simulink subsystem "From_relay_board"  (R2021b)
settings: Solver=VariableStepAuto  StartTime=0.0  StopTime=10.0  RelTol=1e-3
libraries: rti1401lib_dio_type4 x3, rtican x1
settings Model: Creator=tsuyoshi  LastModifiedBy=tsuyoshi

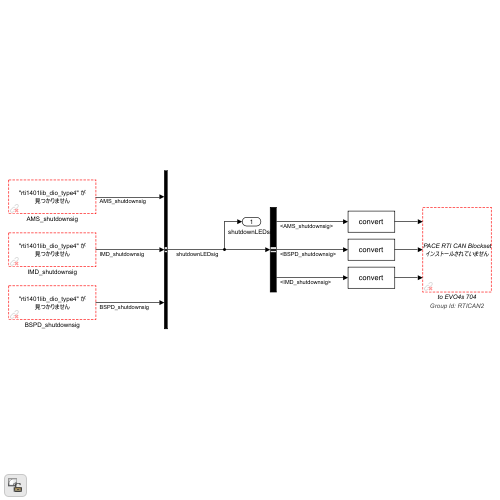
[thumbnail: Simulink's stored preview of the top-level diagram]
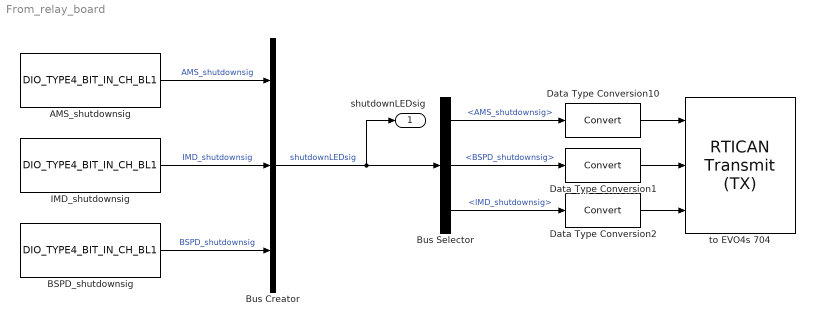
== system From_relay_board ==
  AMS_shutdownsig : rti1401lib_dio_type4/DIO_TYPE4_BIT_IN_CH_BL1  DSProperties=struct('RTI',struct('Version',uint32(1),'BlockType',struct('isSLSource',uint8(1),'isSLSink',uint8(0),'isHWSource',uint8(1),'isHWSink',uint8(0),'isSetup',uint8(0),'isInline',uint8(1),'isNonInline',uint8(0),'isInterrupt',uint8(0),'isChannelwise',uint8(1)),'IOBoardType',{{'DS1401','STD','DIOT4'}},'UnitType','BIT','Identifier','BITINCH','DialogType','ML','BlockSet','NONE','SlaveProcessor','NONE'))  RTIBlockInterface=struct('OutputPortsWidth',int32(1),'OutputPortsDataType',{{'SS_BOOLEAN'}},'OutputPortsActive',1,'OutputPortsName',{{'Out'}},'BlockDisplay',{{['DIO TP4 BIT IN\n Channelwise\nModule: 1\nPort: 1\nChannel: 5'],'center'}},'IconTransparency','on','InitLevel',3,'DialogFcn','rti1401stddiot4bitinchgui','BlockName',struct('Token',{{'DIO_TYPE4_BIT_IN_CH_BL1'}}))  RTIBlockParameters=struct('ModuleNo',{{1,'OFF',[1 16]}},'PortNo',{{1,'OFF',[1 2]}},'ChannelNo',{{5,'OFF',[1 16]}},'TLCFileName',{{'rti1401dio_t4_bit_in_ch','OFF',[]}},'EnableInterrupt',{{0,'OFF',[0 1]}},'TriggerEdgeType',{{1,'OFF',[1 3]}})  RTISFcnParameters=struct('ModuleNo','int32','PortNo','int16','ChannelNo','int16','TLCFileName','char','EnableInterrupt','int16','TriggerEdgeType','int32')  RTIBlockParaDefault=struct('ModuleNo',1,'PortNo',1,'ChannelNo',1,'TLCFileName','rti1401dio_t4_bit_in_ch','EnableInterrupt',0,'TriggerEdgeType',1)
  BSPD_shutdownsig : rti1401lib_dio_type4/DIO_TYPE4_BIT_IN_CH_BL1  DSProperties=struct('RTI',struct('Version',uint32(1),'BlockType',struct('isSLSource',uint8(1),'isSLSink',uint8(0),'isHWSource',uint8(1),'isHWSink',uint8(0),'isSetup',uint8(0),'isInline',uint8(1),'isNonInline',uint8(0),'isInterrupt',uint8(0),'isChannelwise',uint8(1)),'IOBoardType',{{'DS1401','STD','DIOT4'}},'UnitType','BIT','Identifier','BITINCH','DialogType','ML','BlockSet','NONE','SlaveProcessor','NONE'))  RTIBlockInterface=struct('OutputPortsWidth',int32(1),'OutputPortsDataType',{{'SS_BOOLEAN'}},'OutputPortsActive',1,'OutputPortsName',{{'Out'}},'BlockDisplay',{{['DIO TP4 BIT IN\n Channelwise\nModule: 1\nPort: 1\nChannel: 15'],'center'}},'IconTransparency','on','InitLevel',3,'DialogFcn','rti1401stddiot4bitinchgui','BlockName',struct('Token',{{'DIO_TYPE4_BIT_IN_CH_BL1'}}))  RTIBlockParameters=struct('ModuleNo',{{1,'OFF',[1 16]}},'PortNo',{{1,'OFF',[1 2]}},'ChannelNo',{{15,'OFF',[1 16]}},'TLCFileName',{{'rti1401dio_t4_bit_in_ch','OFF',[]}},'EnableInterrupt',{{0,'OFF',[0 1]}},'TriggerEdgeType',{{1,'OFF',[1 3]}})  RTISFcnParameters=struct('ModuleNo','int32','PortNo','int16','ChannelNo','int16','TLCFileName','char','EnableInterrupt','int16','TriggerEdgeType','int32')  RTIBlockParaDefault=struct('ModuleNo',1,'PortNo',1,'ChannelNo',1,'TLCFileName','rti1401dio_t4_bit_in_ch','EnableInterrupt',0,'TriggerEdgeType',1)
  Bus Creator : BusCreator  Inputs=3
  Bus Selector : BusSelector  OutputSignals=AMS_shutdownsig,BSPD_shutdownsig,IMD_shutdownsig
  Data Type Conversion1 : DataTypeConversion
  Data Type Conversion10 : DataTypeConversion
  Data Type Conversion2 : DataTypeConversion
  IMD_shutdownsig : rti1401lib_dio_type4/DIO_TYPE4_BIT_IN_CH_BL1  DSProperties=struct('RTI',struct('Version',uint32(1),'BlockType',struct('isSLSource',uint8(1),'isSLSink',uint8(0),'isHWSource',uint8(1),'isHWSink',uint8(0),'isSetup',uint8(0),'isInline',uint8(1),'isNonInline',uint8(0),'isInterrupt',uint8(0),'isChannelwise',uint8(1)),'IOBoardType',{{'DS1401','STD','DIOT4'}},'UnitType','BIT','Identifier','BITINCH','DialogType','ML','BlockSet','NONE','SlaveProcessor','NONE'))  RTIBlockInterface=struct('OutputPortsWidth',int32(1),'OutputPortsDataType',{{'SS_BOOLEAN'}},'OutputPortsActive',1,'OutputPortsName',{{'Out'}},'BlockDisplay',{{['DIO TP4 BIT IN\n Channelwise\nModule: 1\nPort: 1\nChannel: 10'],'center'}},'IconTransparency','on','InitLevel',3,'DialogFcn','rti1401stddiot4bitinchgui','BlockName',struct('Token',{{'DIO_TYPE4_BIT_IN_CH_BL1'}}))  RTIBlockParameters=struct('ModuleNo',{{1,'OFF',[1 16]}},'PortNo',{{1,'OFF',[1 2]}},'ChannelNo',{{10,'OFF',[1 16]}},'TLCFileName',{{'rti1401dio_t4_bit_in_ch','OFF',[]}},'EnableInterrupt',{{0,'OFF',[0 1]}},'TriggerEdgeType',{{1,'OFF',[1 3]}})  RTISFcnParameters=struct('ModuleNo','int32','PortNo','int16','ChannelNo','int16','TLCFileName','char','EnableInterrupt','int16','TriggerEdgeType','int32')  RTIBlockParaDefault=struct('ModuleNo',1,'PortNo',1,'ChannelNo',1,'TLCFileName','rti1401dio_t4_bit_in_ch','EnableInterrupt',0,'TriggerEdgeType',1)
  to EVO4s 704 : rtican/RTICAN Transmit (TX)   Reserved1=[]  Reserved2=[]  Reserved3=[]  Reserved4=[]  SfcnMessage=[]  Msg_Struct=[]  BoardTypeNo=[]  BoardNo=[]  ChannelNo=[]  Parameters=[]  DialogFcn=[]  UnitName=[]  Revision=[]  UnitValues=[]  DSProperties=struct('RTI',struct('Version',uint32(5),'BlockType',struct('isSLSource',uint8(1),'isSLSink',uint8(1),'isHWSource',uint8(0),'isHWSink',uint8(0),'isSetup',uint8(0),'isInline',uint8(1),'isNonInline',uint8(0),'isInterrupt',uint8(0),'isChannelwise',uint8(0)),'IOBoardType','RTICAN','UnitType','MESSAGE','Identifier','TX','DialogType','MSVC','BlockSet','RTICAN','SlaveProcessor','CAN'))  RTIBlockInterface=struct('InputPortsWidth',int32([1 1 1]),'InputPortsActive',[1 1 1],'InputPortsName',{{'AMS_shutdownsig','BSPD_shutdownsig','IMD_shutdownsig'}},'InputPortsDataType',{{'SS_DOUBLE','SS_DOUBLE','SS_DOUBLE'}},'OutputPortsWidth',int32(0),'OutputPortsActive',0,'OutputPortsName',{{''}},'DialogFcn','rtican_message_interface_gui','BlockDisplay',{{'','center'}},'IconTransparency','on','InitLevel',3,'BlockName',struct('Token',{{'CAN_TYPE','_TX_M','_C'}},'BlockParam',{{'BoardTypeNo','BoardNo','ChannelNo'}}),'SampleTime',{{-1}},'TriggerPort',{{'none'}},'EnablePort',{{'none'}})  RTIBlockParameters=struct('BoardTypeNo',{{1,'OFF',[]}},'BoardNo',{{1,'ON',[1 16]}},'ChannelNo',{{2,'ON',[1 2]}},'Parameters',{{struct('DataFileSupport',struct('DataFileSelectedMaster',0,'DataFileSelectedLocal',0,'DataFileName',['<no datafile support>|'],'DataFileDate','','SelectedFile',['<no file selected>']),'Options',struct('StatusSelected',0,'TimeSelected',0,'DeltaTimeSelected',0,'DelayTimeSelected',0,'DelayTimeTXCommandSelected',0,'EncodeSetUnusedBitsToOne',0,'EnableMsgLoopback',0,'TriggerPort',struct('Selected',0,'TriggerType',0),'EnablePortSelected',0,'SignalOnPortnameSelected',1,'UserCoding',struct('Selected',0,'InterfaceFile','UserEncodingFile','FcnName','UserEncodeFcn','InportSelected',0,'InportWidth',1,'OutportSelected',0,'OutportWidth',1),'TerminationMsg',struct('Selected',0,'Byte0_7','0'),'InitialMsg',struct('Selected',0,'Byte0_7','0')),'Message',struct('MsgOnBlocknameSelected',0,'MsgName','EVO4s005','MsgIdFormat',0,'MsgId',1796,'MsgLength',8,'NumSignals',3,'SampleTime',-1,'StartTime',struct('Selected',0,'Value',0),'AutoRepeatTime',struct('Selected',0,'Value',0.1),'Timeout',struct('Selected',0,'Value',0.1),'DelayTime',struct('Selected',0,'Value',0.1),'Signal',struct('SgnName',{'AMS_shutdownsig','BSPD_shutdownsig','IMD_shutdownsig'},'SgnStartBit',{0,1,2},'SgnLength',{1,1,1},'SgnType',{0,0,0},'ModeValue',{-1,-1,-1},'DataType',{1,1,1},'ByteLayout',{1,1,1},'Factor',{1,1,1},'Offset',{0,0,0},'SgnComment',{{''},{''},{''}},'SgnUnit',{'','',''},'Min',{0,0,0},'Max',{0,0,0},'SLDataType',{'SS_DOUBLE','SS_DOUBLE','SS_DOUBLE'}),'MsgIdNumFormat',1,'MsgComment',{{''}}),'Version',1.2,'general',struct('isFromLib',0)),'OFF',[]}},'GroupId',{{struct('Group',{{'RTICAN'}},'No',2,'Behavior',{{'NAMECHANGE'}},'BlockType',{{'SINK'}},'NameChangeFlag',0),'OFF',[]}},'SFcnRTICANMessage',{{struct('MsgType','TX','SFcnPortType','Scalar','MsgName','EVO4s005','MsgIdFormat','STD','MsgId',1796,'MsgLength',8,'NumSignals',3,'SampleTime',-1,'StartTime',struct('Selected','no','Value',0),'AutoRepeatTime',struct('Selected','no','Value',0.1),'Timeout',struct('Selected','no','Value',0.1),'Signal',struct('SgnName',{'AMS_shutdownsig','BSPD_shutdownsig','IMD_shutdownsig'},'SgnStartBit',{0,1,2},'SgnLength',{1,1,1},'SgnType',{'standard','standard','standard'},'ModeValue',{-1,-1,-1},'DataType',{['signed int'],['signed int'],['signed int']},'ByteLayout',{['big endian'],['big endian'],['big endian']},'Factor',{1,1,1},'Offset',{0,0,0},'SLDataType',{'SS_DOUBLE','SS_DOUBLE','SS_DOUBLE'}),'StatusSelected','no','TimeSelected','no','DeltaTimeSelected','no','DelayTimeSelected','no','DelayTimeTXCommandSelected','no','EncodeSetUnusedBitsToOne','no','EnableMsgLoopback','no','TriggerPort',struct('Selected','no','TriggerType',0),'EnablePortSelected','no','UserCoding',struct('Selected','no','InterfaceFile','UserEncodingFile','FcnName','UserEncodeFcn','InportSelected','no','InportWidth',1,'OutportSelected','no','OutportWidth',1),'TerminationMsg',struct('Selected','no','Byte0','0x00','Byte1','0x00','Byte2','0x00','Byte3','0x00','Byte4','0x00','Byte5','0x00','Byte6','0x00','Byte7','0x00'),'InitialMsg',struct('Selected','no','Byte0','0x00','Byte1','0x00','Byte2','0x00','Byte3','0x00','Byte4','0x00','Byte5','0x00','Byte6','0x00','Byte7','0x00'),'BoardType','DS1','BoardNo',1,'ControllerNo',2),'OFF',[]}},'TLCFileName',{{'rtican_tx_message','OFF',[]}})  RTISFcnParameters=struct('SFcnRTICANMessage','struct','TLCFileName','char')  RTIBlockParaDefault=struct('BoardTypeNo',4302,'BoardNo',1,'ChannelNo',1,'Parameters',struct('DataFileSupport',struct('DataFileSelectedMaster',0,'DataFileSelectedLocal',0,'DataFileName','','DataFileDate','','SelectedFile',['<no file selected>']),'Options',struct('StatusSelected',1,'TimeSelected',1,'DeltaTimeSelected',1,'DelayTimeSelected',1,'DelayTimeTXCommandSelected',0,'EncodeSetUnusedBitsToOne',0,'EnableMsgLoopback',0,'TriggerPort',struct('Selected',0,'TriggerType','rising'),'EnablePortSelected',0,'SignalOnPortnameSelected',1,'UserCoding',struct('Selected',0,'InterfaceFile','UserEncodingFile','FcnName','UserEncodeFcn','InportSelected',0,'InportWidth',1,'OutportSelected',0,'OutportWidth',1),'TerminationMsg',struct('Selected',0,'Byte0_7','0'),'InitialMsg',struct('Selected',0,'Byte0_7','0')),'Message',struct('MsgOnBlocknameSelected',0,'MsgName',['TX Message'],'MsgIdFormat',0,'MsgId',100,'MsgLength',8,'NumSignals',1,'SampleTime',-1,'StartTime',struct('Selected',0,'Value',0),'AutoRepeatTime',struct('Selected',0,'Value',0.1),'Timeout',struct('Selected',0,'Value',0.1),'DelayTime',struct('Selected',0,'Value',0.1),'Signal',struct('SgnName',['TX signal'],'SgnStartBit',0,'SgnLength',8,'SgnType',0,'ModeValue',-1,'DataType',0,'SLDataType','SS_DOUBLE','ByteLayout',0,'Factor',1,'Offset',0,'Min',0,'Max',255,'SgnComment',{{}},'SgnUnit',''),'MsgIdNumFormat',0,'MsgComment',{{''}}),'Version',1.2,'general',struct('isFromLib',1)),'GroupId',struct('Group',{{'RTICAN'}},'No',1,'Behavior',{{'NAMECHANGE'}},'BlockType',{{'SINK'}},'NameChangeFlag',0),'SFcnRTICANMessage',struct('MsgType','TX','MsgName',['TX Message'],'MsgIdFormat','STD','MsgId',100,'MsgLength',2,'NumSignals',1,'SampleTime',-1,'StartTime',struct('Selected','no','Value',0),'AutoRepeatTime',struct('Selected','no','Value',0.1),'Timeout',struct('Selected','no','Value',0.1),'DelayTime',struct('Selected','no','Value',0.1),'Signal',struct('SgnName',['TX signal'],'SgnStartBit',0,'SgnLength',8,'SgnType','standard','ModeValue',-1,'DataType',['unsigned int'],'ByteLayout',['little endian'],'SLDataType','SS_DOUBLE','Factor',1,'Offset',0),'StatusSelected','yes','TimeSelected','yes','DeltaTimeSelected','yes','DelayTimeSelected','yes','EnablePortSelected','no','EnableMsgLoopback','no','DelayTimeTXCommandSelected','no','EncodeSetUnusedBitsToOne','no','UserCoding',struct('Selected','no','InterfaceFile','UserDecodingFile','FcnName','UserDecodeFcn','InportSelected','no','InportWidth',1,'OutportSelected','no','OutportWidth',1),'TerminationMsg',struct('Selected','no','Byte0','0x00','Byte1','0x00','Byte2','0x00','Byte3','0x00','Byte4','0x00','Byte5','0x00','Byte6','0x00','Byte7','0x00'),'InitialMsg',struct('Selected','no','Byte0','0x00','Byte1','0x00','Byte2','0x00','Byte3','0x00','Byte4','0x00','Byte5','0x00','Byte6','0x00','Byte7','0x00'),'TriggerPort',struct('Selected','no','TriggerType','rising'),'BoardType','DS4302','BoardNo',1,'ControllerNo',1,'SFcnPortType','Scalar'),'TLCFileName','rtican_tx_message')
      settings: AttributesFormatString=Group Id: RTICAN2\n  SourceProductName=dSPACE RTI CAN Blockset
  shutdownLEDsig : Outport
  wires:
  AMS_shutdownsig/1 -> Bus Creator/1  "AMS_shutdownsig"
  IMD_shutdownsig/1 -> Bus Creator/2  "IMD_shutdownsig"
  BSPD_shutdownsig/1 -> Bus Creator/3  "BSPD_shutdownsig"
  Bus Creator/1 -> shutdownLEDsig/1, Bus Selector/1  "shutdownLEDsig"
  Bus Selector/2 -> Data Type Conversion1/1  "<BSPD_shutdownsig>"
  Bus Selector/1 -> Data Type Conversion10/1  "<AMS_shutdownsig>"
  Data Type Conversion10/1 -> to EVO4s 704/1
  Data Type Conversion2/1 -> to EVO4s 704/3
  Data Type Conversion1/1 -> to EVO4s 704/2
  Bus Selector/3 -> Data Type Conversion2/1  "<IMD_shutdownsig>"
